simulink model "L9T1_Gridconnected_HysteresisControlH_BridgeInverterUni"  (R2021a)
settings: Solver=VariableStepAuto  StartTime=0.0  StopTime=inf  RelTol=1e-3
undefined symbols (not defined in the file): Acid, Lead
libraries: spsIGBTDiodeLib x6, spsSeriesRLCBranchLib x3, spsVoltageMeasurementLib x3, spsCurrentMeasurementLib x2, spsACVoltageSourceLib x1, spsBatteryLib x1, pid_lib x1, spsPLLLib x1, spsPWMGeneratorDCDCLib x1, spspowerguiLib x1
settings Model: Creator=hp  LastModifiedBy=hp

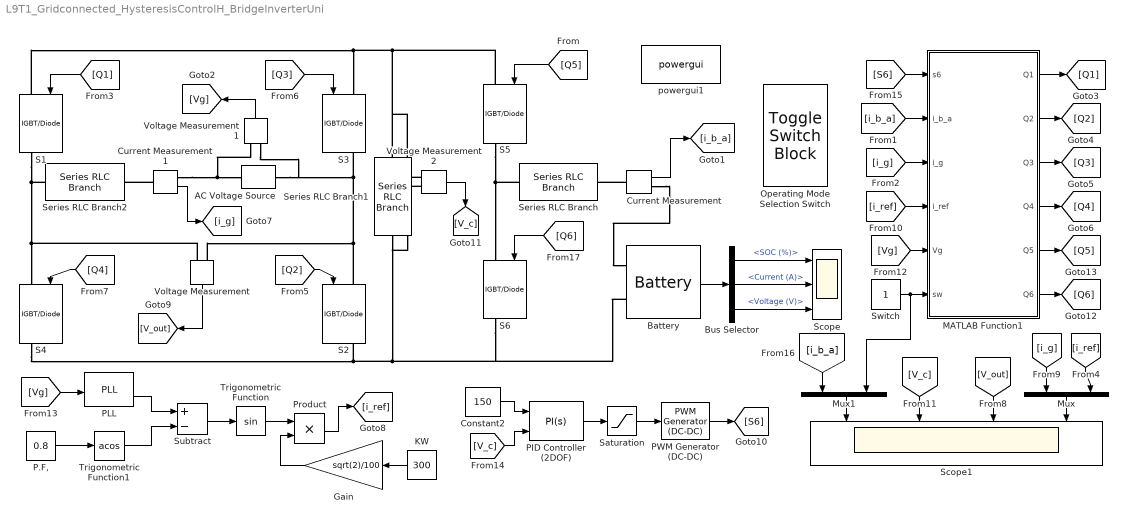
== system L9T1_Gridconnected_HysteresisControlH_BridgeInverterUni ==
  AC Voltage Source : spsACVoltageSourceLib/AC Voltage Source  Amplitude=100*sqrt(2)  Phase=0  Frequency=50  SampleTime=0  Measurements=None  BusType=swing  Pref=10e3  Qref=0  Qmin=-inf  Qmax=+inf
  Battery : spsBatteryLib/Battery  BatType=Lead-Acid  ShowTempParam=off  ThermalPreset=no  ShowAgeParam=off  NomV=60  NomQ=5.4  SOC=70  Batt_Tr=30  PresetModel=on  MaxQ=5.625  MinV=45  FullV=65.3289  Dis_rate=1.08  R=0.11111  Normal_OP=1.6755  expZone="[61.0855        0.018]"  current=[6.5 13 32.5]  Units=Time  Tci=20  NomT=20  T2=-30  MaxQ2=4.8  FullV2=7.1  Normal_OP2=5.655  expZone2="[6.58           1]"  Rca=0.6  ti=2000  Dp=0  Neq0=0  Tsim=1e6  Ta1=25  Qeol=5.4*0.9  Reol=0.013333*1.2  Char_age=[2.3478, 3]  Dis_age=[2.3478, 10]  N1=1500  N2=10500  N3=1000  N4=1400  Ta2=45  N5=950
  Bus Selector : BusSelector  OutputSignals=SOC (%),Current (A),Voltage (V)
  Constant2 : Constant  Value=150
  Current Measurement : spsCurrentMeasurementLib/Current Measurement  PhasorSimulation=off  OutputType=Complex  PSBequivalent=0
  Current Measurement1 : spsCurrentMeasurementLib/Current Measurement  PhasorSimulation=off  OutputType=Complex  PSBequivalent=0
  Gain : Gain  Gain=sqrt(2)/100
  KW : Constant  Value=300
  MATLAB Function1 : MATLAB Function  TreatAsAtomicUnit=on
  Mux : Mux  Inputs=2
  Mux1 : Mux  Inputs=2
  Operating Mode Selection Switch : ToggleSwitchBlock
      settings: Values={{'Off', 'On'}, [1 2]}
  P.F, : Constant  Value=0.8
  PID Controller (2DOF) : pid_lib/PID Controller (2DOF)  Controller=PI  Form=Parallel  TimeDomain=Continuous-time  UseExternalTs=off  SampleTime=-1  IntegratorMethod=Forward Euler  FilterMethod=Forward Euler  ControllerParametersSource=internal  P=0.1  I=0.01  D=0  UseFilter=on  N=100  b=1  c=1  TunerSelectOption=Transfer Function Based (PID Tuner App)  InitialConditionSource=internal  InitialConditionForIntegrator=0  InitialConditionForFilter=0  DifferentiatorICPrevScaledInput=0  ExternalReset=none  TrackingMode=off  Kt=1  LimitOutput=off  SatLimitsSource=internal  UpperSaturationLimit=inf  LowerSaturationLimit=-inf  LinearizeAsGain=on  AntiWindupMode=none  Kb=1  POutMin=[]  POutMax=[]  IOutMin=[]  IOutMax=[]  DOutMin=[]  DOutMax=[]  NOutMin=[]  NOutMax=[]  bOutMin=[]  bOutMax=[]  cOutMin=[]  cOutMax=[]  SumOutMin=[]  SumOutMax=[]  SaturationOutMin=[]  SaturationOutMax=[]  PParamMin=[]  PParamMax=[]  IParamMin=[]  IParamMax=[]  DParamMin=[]  DParamMax=[]  NParamMin=[]  NParamMax=[]  bParamMin=[]  bParamMax=[]  cParamMin=[]  cParamMax=[]  KbParamMin=[]  KbParamMax=[]  KtParamMin=[]  KtParamMax=[]  KbOutMin=[]  KbOutMax=[]  KtOutMin=[]  KtOutMax=[]  IntegratorOutMin=[]  IntegratorOutMax=[]  FilterOutMin=[]  FilterOutMax=[]  SumI1OutMin=[]  SumI1OutMax=[]  SumI2OutMin=[]  SumI2OutMax=[]  SumI3OutMin=[]  SumI3OutMax=[]  SumI4OutMin=[]  SumI4OutMax=[]  SumDOutMin=[]  SumDOutMax=[]  Sum1OutMin=[]  Sum1OutMax=[]  Sum2OutMin=[]  Sum2OutMax=[]  Sum3OutMin=[]  Sum3OutMax=[]  DifferentiatorOutMin=[]  DifferentiatorOutMax=[]  FilterDiffOutCoefMin=[]  FilterDiffOutCoefMax=[]  ReciprocalOutMin=[]  ReciprocalOutMax=[]  SumDenOutMin=[]  SumDenOutMax=[]  SumNumOutMin=[]  SumNumOutMax=[]  DivideOutMin=[]  DivideOutMax=[]  UdiffTsProdOutMin=[]  UdiffTsProdOutMax=[]  NTsProdOutMin=[]  NTsProdOutMax=[]  UintegralTsProdOutMin=[]  UintegralTsProdOutMax=[]  UngainTsProdOutMin=[]  UngainTsProdOutMax=[]  IntegratorContinuousStateAttributes=''  IntegratorStateMustResolveToSignalObject=off  IntegratorRTWStateStorageClass=Auto  FilterContinuousStateAttributes=''  FilterStateMustResolveToSignalObject=off  FilterRTWStateStorageClass=Auto  ParallelPVariant=InternalParameters  IdealPVariant=Disabled  IVariant=InternalParameters  DVariant=Disabled  bVariant=InternalParameters  cVariant=Disabled  IntegratorVariant=Continuous  SatVariant=Disabled  AWVariant=Passthrough  PCopyVariant=Disabled  TRVariant=Disabled  FdbkBlocksVariant=Forward  IdealPFdbkVariant=Disabled  SatFdbkVariant=Disabled  DerivativeFilterVariant=Disabled  NVariant=Disabled  NCopyVariant=Disabled_SignalSpec  FilterICVariant=Disabled  IntegratorICVariant=InternalICs  ExternalResetVariant=Disabled  TRSumVariant=Passthrough  SumFdbkVariant=Disabled  SumVariant=Sum_PI  TsampFilterVariant=InternalTs  TsampNgainVariant=Passthrough  TsampIntegralVariant=Passthrough  ExternalSaturationOutDataTypeStr=Inherit: Same as second input
      settings: SourceProductBaseCode=SL
  PLL : spsPLLLib/PLL  Fmin=45  Par_Init=[0, 50]  ParK=[180, 3200, 1]  TcD=1e-4  MaxRateChangeFreq=12  FilterCutOffFreq=25  Ts=0  AGC=on
      settings: SourceProductBaseCode=PS
  PWM Generator (DC-DC) : spsPWMGeneratorDCDCLib/PWM Generator (DC-DC)  Fsw=5000  Ts=0
  Product : Product
  S{1..6} (6 alike) : spsIGBTDiodeLib/IGBT//Diode  Ron=1e-3  Rs=1e5  Cs=inf  Measurements=on
  Saturation : Saturate  LowerLimit=0
  Scope : Scope  NumInputPorts=3
  Scope1 : Scope  NumInputPorts=4
  Series RLC Branch : spsSeriesRLCBranchLib/Series RLC Branch  LConnTagsString=__new0  RConnTagsString=__new0  BranchType=RL  Resistance=0.1  Inductance=5e-3  SetiL0=off  InitialCurrent=0  Capacitance=1e-6  Setx0=off  InitialVoltage=0  Measurements=None
  Series RLC Branch1 : spsSeriesRLCBranchLib/Series RLC Branch  LConnTagsString=__new0  RConnTagsString=__new0  BranchType=C  Resistance=0.1  Inductance=5e-3  SetiL0=off  InitialCurrent=0  Capacitance=1000e-6  Setx0=off  InitialVoltage=0  Measurements=None
  Series RLC Branch2 : spsSeriesRLCBranchLib/Series RLC Branch  LConnTagsString=__new0  RConnTagsString=__new0  BranchType=RL  Resistance=0.1  Inductance=5e-3  SetiL0=off  InitialCurrent=0  Capacitance=1e-6  Setx0=off  InitialVoltage=0  Measurements=None
  Subtract : Sum  Inputs=+-
  Switch : Constant
  Trigonometric Function : Trigonometry
  Trigonometric Function1 : Trigonometry  Operator=acos
  Voltage Measurement : spsVoltageMeasurementLib/Voltage Measurement  PhasorSimulation=off  OutputType=Complex  PSBequivalent=0
  Voltage Measurement1 : spsVoltageMeasurementLib/Voltage Measurement  PhasorSimulation=off  OutputType=Complex  PSBequivalent=0
  Voltage Measurement2 : spsVoltageMeasurementLib/Voltage Measurement  PhasorSimulation=off  OutputType=Complex  PSBequivalent=0
  powergui1 : spspowerguiLib/powergui  Priority=1  SimulationMode=Discrete  SampleTime=50e-6  frequency=60  Iterations=50  frequencyindice=50  Pbase=100e6  ErrMax=1e-4  UnitsV=kV  UnitsW=MW  buscounter=0  FunctionMessages=off  echomessages=off  EnableUseOfTLC=off  CurrentSourceSwitches=off  DisableSnubberDevices=off  DisableRonSwitches=off  DisableVfSwitches=off  DisplayEquations=off  AutomaticDiscreteSolvers=off  SolverType=Tustin/Backward Euler (TBE)  Interpol=off  ExternalGateDelay=off  methode=off  Ts=100  x0status=blocks  SPID=on  SwTol=0  HookPort=off  NonlinearTolerance=1e-4  nMaxIteration=100  ContinueOnMaxIteration=off  RestoreLinks=warning  ResistiveCurrentMeasurement=off  Frange=[0:2:500]  Ylog=off  Xlog=on  ShowGrid=off  save=off  variable=ZData  structure=0  ZoomFFT=off  StartTime=0.0  cycles=1  DisplayStyle=1  fundamental=60  FreqAxis=off  MaxFrequency=1000  frequencyindicesteady=1  RmsSteady=1  display=off
  wires:
  [Q6] -> S6/1
  [Q5] -> S5/1
  Current Measurement/1 -> [i_b_a]
  Trigonometric Function/1 -> Product/1
  Gain/1 -> Product/2
  P.F,/1 -> Trigonometric Function1/1
  Product/1 -> [i_ref]
  Subtract/1 -> Trigonometric Function/1
  [Vg] -> PLL/1
  MATLAB Function1/3(Q3) -> [Q3]
  KW/1 -> Gain/1
  MATLAB Function1/1(Q1) -> [Q1]
  Trigonometric Function1/1 -> Subtract/2
  MATLAB Function1/4(Q4) -> [Q4]
  MATLAB Function1/2(Q2) -> [Q2]
  PLL/2 -> Subtract/1
  Voltage Measurement1/1 -> [Vg]
  [Q1] -> S1/1
  [Q2] -> S2/1
  [Q3] -> S3/1
  [Q4] -> S4/1
  Current Measurement1/1 -> [i_g]
  Voltage Measurement/1 -> [V_out]
  PWM Generator (DC-DC)/1 -> [S6]
  [V_c] -> PID Controller (2DOF)/2
  Constant2/1 -> PID Controller (2DOF)/1
  Saturation/1 -> PWM Generator (DC-DC)/1
  PID Controller (2DOF)/1 -> Saturation/1
  Voltage Measurement2/1 -> [V_c]
  MATLAB Function1/5(Q5) -> [Q5]
  MATLAB Function1/6(Q6) -> [Q6]
  [i_g] -> MATLAB Function1/3(i_g)
  [i_ref] -> MATLAB Function1/4(i_ref)
  [i_b_a] -> MATLAB Function1/2(i_b_a)
  [Vg] -> MATLAB Function1/5(Vg)
  Mux/1 -> Scope1/4
  [V_out] -> Scope1/3
  [V_c] -> Scope1/2
  [i_g] -> Mux/1
  [i_ref] -> Mux/2
  Battery/1 -> Bus Selector/1
  Bus Selector/1 -> Scope/1  "<SOC (%)>"
  Bus Selector/3 -> Scope/3  "<Voltage (V)>"
  Mux1/1 -> Scope1/1
  [S6] -> MATLAB Function1/1(s6)
  Switch/1 -> MATLAB Function1/6(sw), Mux1/2
  [i_b_a] -> Mux1/1
  Bus Selector/2 -> Scope/2  "<Current (A)>"
  connections:
  S1/RConn1 -- Voltage Measurement/LConn1 -- S4/LConn1 -- Series RLC Branch2/LConn1
  S1/LConn1 -- Series RLC Branch1/LConn1 -- Voltage Measurement2/LConn1 -- S5/LConn1 -- S3/LConn1
  S4/RConn1 -- S2/RConn1 -- S6/RConn1 -- Battery/LConn2 -- Voltage Measurement2/LConn2 -- Series RLC Branch1/RConn1
  S2/LConn1 -- AC Voltage Source/LConn1 -- Voltage Measurement1/LConn2 -- S3/RConn1 -- Voltage Measurement/LConn2
  S5/RConn1 -- Series RLC Branch/LConn1 -- S6/LConn1
  Current Measurement/LConn1 -- Series RLC Branch/RConn1
  Current Measurement/RConn1 -- Battery/LConn1
  Current Measurement1/LConn1 -- Series RLC Branch2/RConn1
  Current Measurement1/RConn1 -- Voltage Measurement1/LConn1 -- AC Voltage Source/RConn1

== matlab function L9T1_Gridconnected_HysteresisControlH_BridgeInverterUni/MATLAB Function1 ==
  settings: updateMethod=DISCRETE
  data: s6 input; i_b_a input; i_g input; i_ref input; Vg input; sw input; Q1 output; Q2 output; Q3 output; Q4 output; Q5 output; Q6 output
function [Q1,Q2,Q3,Q4,Q5,Q6] = fcn(s6,i_b_a,i_g,i_ref,Vg,sw)
persistent S1 S2 S3 S4 S5 S6;
if isempty(S1)
    S1=0;
end
if isempty(S2)
    S2=0;
end
if isempty(S3)
    S3=0;
end
if isempty(S4)
    S4=0;
end
if isempty(S5)
    S5=1;
end
if isempty(S6)
    S6=0;
end
d=0.5;
i_b_ref=5;
e=i_b_a-i_b_ref;
e1=i_g-i_ref;
if  sw==1
    S1=0;   S2=0;   S3=0;   S4=0;   S6=0;
    if e>=d
        S5=0;
    elseif e<=-d
        S5=1;
    else
        S5=S5;
    end
else sw==2
    S6=s6;
    S5=0;
    if Vg>=0
        if e1<=-d
            S1=1;   S2=1;   S3=0;   S4=0;
        elseif e1>=d
            S1=1;   S2=0;   S3=1;   S4=0;
        else
            S1=S1;  S2=S2;  S3=S3;  S4=S4;
        end
    else
        if e1<=-d
            S1=1;   S2=0;   S3=1;   S4=0;
        elseif e1>=d
            S1=0;   S2=0;   S3=1;   S4=1;
        else
            S1=S1;  S2=S2;  S3=S3;  S4=S4;
        end
    end
end
Q1=S1;  Q2=S2;  Q3=S3;  Q4=S4;  Q5=S5;  Q6=S6;
end
